simulink model "abslut125_fixpt16"  (R2021b)
settings: Solver=VariableStepAuto  StartTime=0.0  StopTime=359  RelTol=1e-3
undefined symbols (not defined in the file or in its folder): S, vsva2197, xcvc1902
libraries: hdlBasic x1350, vmcUtilities x1
(part 4 of 8)

== matlab function abslut125_fixpt16/MATLAB Function ==
  data: u input; y output; x input
function y = fcn(u,x)

y = immse(u,x);

== matlab function abslut125_fixpt16/MATLAB Function2 ==
  data: x input; out output; y input
function out = fcn(x,y)
out = sqrt(x.^2 + y.^2);
